simulink model "simulinkCalisma2"  (R2021b)
settings: Solver=VariableStepAuto  StartTime=0.0  StopTime=10.0  RelTol=1e-3
settings Model: Creator=lenovo  LastModifiedBy=lenovo

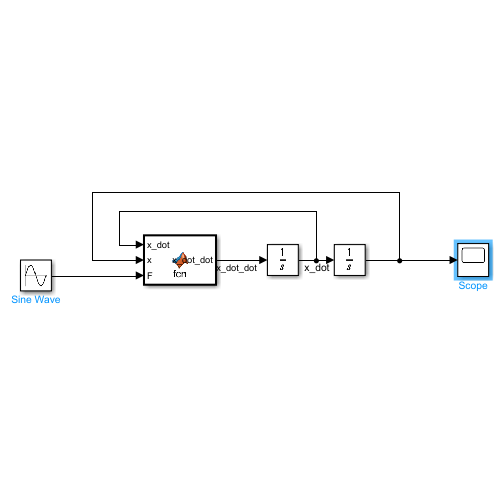
[thumbnail: Simulink's stored preview of the top-level diagram]
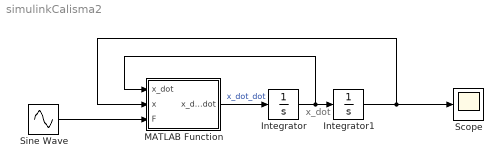
== system simulinkCalisma2 ==
  note: x_dot
  Integrator : Integrator
  Integrator1 : Integrator
  MATLAB Function : MATLAB Function  TreatAsAtomicUnit=on
  Scope : Scope
  Sine Wave : Sin  Frequency=2  SampleTime=0
  wires:
  MATLAB Function/1(x_dot_dot) -> Integrator/1  "x_dot_dot"
  Integrator/1 -> MATLAB Function/1(x_dot), Integrator1/1
  Integrator1/1 -> Scope/1, MATLAB Function/2(x)
  Sine Wave/1 -> MATLAB Function/3(F)

== matlab function simulinkCalisma2/MATLAB Function ==
  data: x_dot input; x_dot_dot output; x input; F input
function x_dot_dot= fcn(x_dot,x,F)
%constant variables 
m=2;    %kg
c=2;   %N/msn
k=2;   %N/m
x_dot_dot=1/m*(F-k*x--c*x_dot);

end
